simulink model "prbs_generator_block_visual_fdbk"  (R2022a)
settings: Solver=VariableStepAuto  StartTime=0.0  StopTime=10.0  RelTol=1e-3
settings Model: Creator=rbme1  LastModifiedBy=rbme1

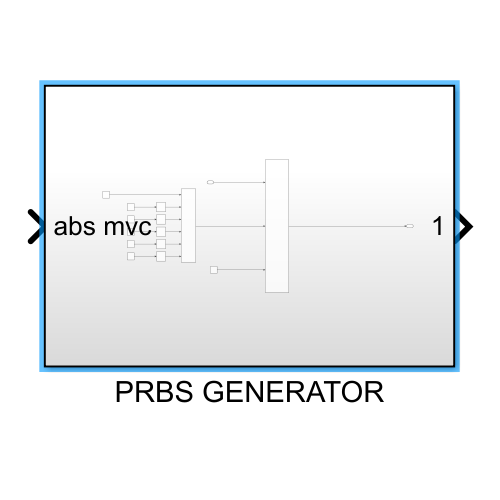
[thumbnail: Simulink's stored preview of the top-level diagram]
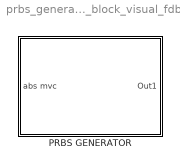
== system prbs_generator_block_visual_fdbk ==
  PRBS GENERATOR : Subsystem

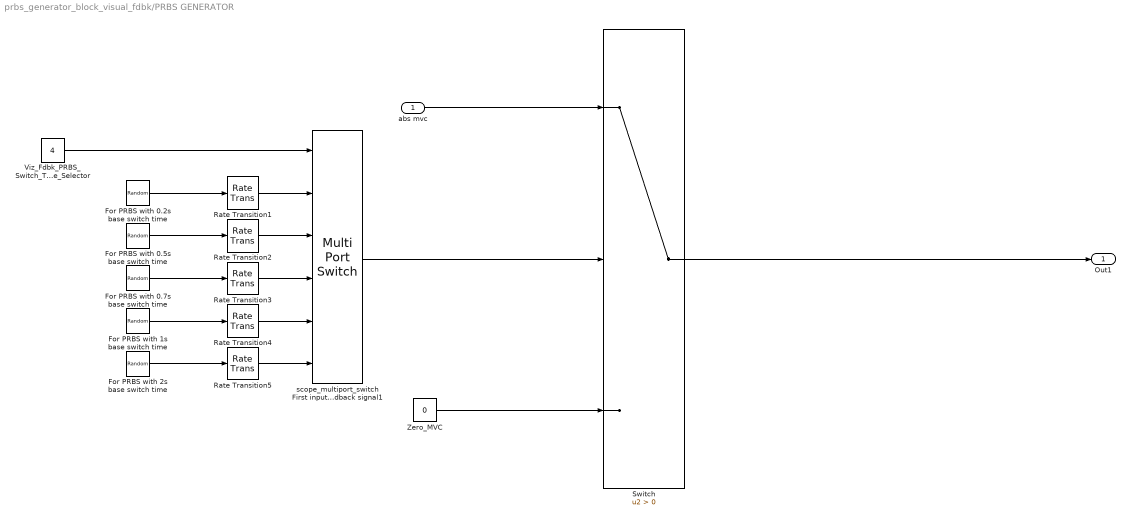
== system prbs_generator_block_visual_fdbk/PRBS GENERATOR ==
  abs mvc : Inport
  For PRBS with 0.2s base switch time : UniformRandomNumber  SampleTime=0.2
  For PRBS with 0.5s base switch time : UniformRandomNumber  SampleTime=0.5
  For PRBS with 0.7s base switch time : UniformRandomNumber  SampleTime=0.7
  For PRBS with 1s base switch time : UniformRandomNumber  SampleTime=1
  For PRBS with 2s base switch time : UniformRandomNumber  SampleTime=2
  Rate Transition{1..5} (5 alike) : RateTransition  OutPortSampleTime=0
  Switch : Switch  Criteria=u2 > Threshold  SaturateOnIntegerOverflow=off  InputSameDT=off
  Viz_Fdbk_PRBS_Switch_Time_Selector : Constant  Value=4
  Zero_MVC : Constant  Value=0
  scope_multiport_switch First input is the desired position Second inpt is the measured position Third input is measured Torque Fourth input is visual feedback signal1 : MultiPortSwitch  Inputs=5  SaturateOnIntegerOverflow=off  InputSameDT=off
  Out1 : Outport
  wires:
  Rate Transition2/1 -> scope_multiport_switch First input is the desired position Second inpt is the measured position Third input is measured Torque Fourth input is visual feedback signal1/3
  For PRBS with 1s base switch time/1 -> Rate Transition4/1
  For PRBS with 0.5s base switch time/1 -> Rate Transition2/1
  For PRBS with 2s base switch time/1 -> Rate Transition5/1
  Rate Transition4/1 -> scope_multiport_switch First input is the desired position Second inpt is the measured position Third input is measured Torque Fourth input is visual feedback signal1/5
  Rate Transition1/1 -> scope_multiport_switch First input is the desired position Second inpt is the measured position Third input is measured Torque Fourth input is visual feedback signal1/2
  Rate Transition5/1 -> scope_multiport_switch First input is the desired position Second inpt is the measured position Third input is measured Torque Fourth input is visual feedback signal1/6
  For PRBS with 0.2s base switch time/1 -> Rate Transition1/1
  Zero_MVC/1 -> Switch/3
  Viz_Fdbk_PRBS_Switch_Time_Selector/1 -> scope_multiport_switch First input is the desired position Second inpt is the measured position Third input is measured Torque Fourth input is visual feedback signal1/1
  For PRBS with 0.7s base switch time/1 -> Rate Transition3/1
  Rate Transition3/1 -> scope_multiport_switch First input is the desired position Second inpt is the measured position Third input is measured Torque Fourth input is visual feedback signal1/4
  scope_multiport_switch First input is the desired position Second inpt is the measured position Third input is measured Torque Fourth input is visual feedback signal1/1 -> Switch/2
  Switch/1 -> Out1/1
  abs mvc/1 -> Switch/1
